simulink model "MagnetoShield_PolePlacement_DUE"  (R2019a)
settings: Solver=FixedStepAuto  StartTime=0.0  StopTime=15  RelTol=1e-3  EnableMultiTasking=on
undefined symbols (not defined in the file): A, B, C, DiscIntNeverNeededParam, i0, K, L, sigbuilder_block, Ts, u0, y0
libraries: MagnetoLibrary x3
settings Model: SimulationMode=external  ExtModeTrigDuration=2  Creator=jakub  LastModifiedBy=jakub
settings OptimizationCC: EnhancedBackFolding=on  PassReuseOutputArgsAs=Individual arguments  MaxStackSize=64  OptimizeBlockOrder=speed  DifferentSizesBufferReuse=on  OptimizationCustomize=off
settings DebuggingCC: ParameterTunabilityLossMsg=error
settings HardwareCC: ProdBitPerPointer=32  ProdBitPerSizeT=32  ProdBitPerPtrDiffT=32  ProdLargestAtomicInteger=Long  ProdLargestAtomicFloat=Double  ProdWordSize=32  ProdHWDeviceType=ARM Compatible->ARM Cortex
settings SFSimCC: MATLABDynamicMemAlloc=off
settings RTWCC: SystemTargetFile=ert.tlc  HardwareBoard=Arduino Due  TLCOptions=-aInlineSetEventsForThisBaseRateFcn=TLC_FALSE -aSuppressMultiTaskScheduler=TLC_FALSE -aRateBasedStepFcn=1  TemplateMakefile=ert_default_tmf  GenerateReport=on  Toolchain=Arduino ARM  BuildConfiguration=Faster Runs  IncludeHyperlinkInReport=on  LaunchReport=on  GenerateTraceInfo=on  GenerateTraceReport=on  GenerateTraceReportSl=on  GenerateTraceReportSf=on  GenerateTraceReportEml=on
settings CodeAppCC: ForceParamTrailComments=on  IgnoreCustomStorageClasses=off  OperatorAnnotations=on  SimulinkDataObjDesc=on  SFDataObjDesc=on  InsertBlockDesc=on
settings ERTTargetCC: SupportContinuousTime=on  SupportVariableSizeSignals=on  ExtModeStaticAllocSize=24576

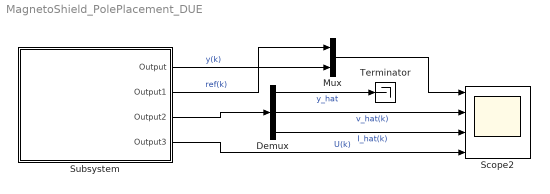
== system MagnetoShield_PolePlacement_DUE ==
  Demux : Demux  Outputs=3
  Mux : Mux  Inputs=2
  Scope2 : Scope  NumInputPorts=4
  Subsystem : Subsystem
  Terminator : Terminator
  wires:
  Subsystem/2(Output1) -> Mux/1  "ref(k)"
  Subsystem/1(Output) -> Mux/2  "y(k)"
  Subsystem/3(Output2) -> Demux/1
  Subsystem/4(Output3) -> Scope2/4  "U(k)"
  Demux/2 -> Scope2/2  "v_hat(k)"
  Demux/3 -> Scope2/3  "I_hat(k)"
  Mux/1 -> Scope2/1
  Demux/1 -> Terminator/1  "y_hat"

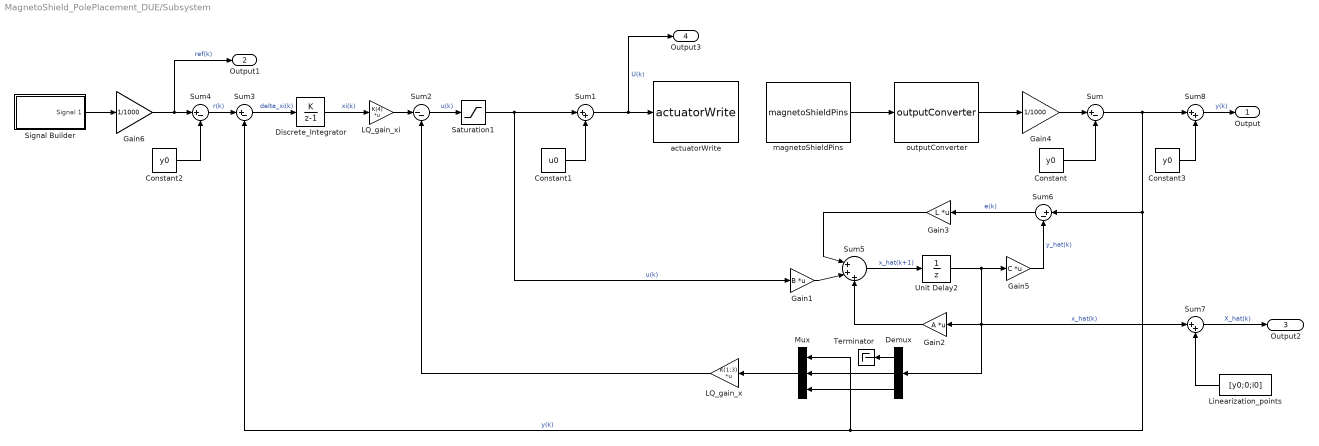
== system MagnetoShield_PolePlacement_DUE/Subsystem ==
  Constant : Constant  Value=y0
  Constant1 : Constant  Value=u0
  Constant2 : Constant  Value=y0
  Constant3 : Constant  Value=y0
  Demux : Demux  Outputs=3
  Discrete_Integrator : DiscreteIntegrator  IntegratorMethod=Accumulation: Forward Euler  SampleTime=Ts  UpperSaturationLimit=1  LowerSaturationLimit=-1  ICPrevOutput=DiscIntNeverNeededParam  ICPrevScaledInput=DiscIntNeverNeededParam
  Gain1 : Gain  Gain=B  Multiplication=Matrix(K*u)
  Gain2 : Gain  Gain=A  Multiplication=Matrix(K*u)
  Gain3 : Gain  Gain=L  Multiplication=Matrix(K*u)
  Gain4 : Gain  Gain=1/1000
  Gain5 : Gain  Gain=C  Multiplication=Matrix(K*u)
  Gain6 : Gain  Gain=1/1000
  LQ_gain_x : Gain  Gain=K(1:3)  Multiplication=Matrix(K*u)
  LQ_gain_xi : Gain  Gain=K(4)  Multiplication=Matrix(K*u)
  Linearization_points : Constant  Value=[y0;0;i0]
  Mux : Mux  Inputs=3
  Saturation1 : Saturate  UpperLimit=10-u0  LowerLimit=0-u0
  Signal Builder : Subsystem  Tag=STV Subsys  LoadFcn=sigbuilder_block('load');  StartFcn=sigbuilder_block('start');  StopFcn=sigbuilder_block('stop');  ClipboardFcn=sigbuilder_block('clipboard');  mask(Sigbuilder block){tuvar=[0:10]}
      mask help: Simulink:masks:SigbuilderBlock_MD
      mask init:
      | if ~strcmp(get_param(bdroot(gcbh),'SimulationStatus'),'stopped') tuvar = sigbuilder_block('maskInit'); end
      settings: CopyFcn=sigbuilder_block('copy');  DeleteFcn=sigbuilder_block('delete');  ModelCloseFcn=sigbuilder_block('modelClose');  PreSaveFcn=sigbuilder_block('preSave');  PauseFcn=sigbuilder_block('pause');  ContinueFcn=sigbuilder_block('continue');  NameChangeFcn=sigbuilder_block('namechange');  OpenFcn=sigbuilder_block('open',[434.4 169.8 550.8 400.2 ]);  CloseFcn=sigbuilder_block('close');
      mask Display: plot(0, 0, 100, 100,[2, 2, 32, 32, 2], [68, 8, 8, 68, 68],[32, 2], [38, 38], [32, 19, 2],[53, 60, 44], [32, 17, 17, 2],[16, 16, 31, 31]);txt = getActiveGroup(gcbh);text(2, 100, txt,'verticalAlignment', 'top');
  Sum{,3..4,6} (4 alike) : Sum  Inputs=|+-
  Sum1 : Sum  Inputs=|++
  Sum2 : Sum  Inputs=|--
  Sum5 : Sum  Inputs=|+++
  Sum7 : Sum  Inputs=|++
  Sum8 : Sum  Inputs=|++
  Terminator : Terminator
  Unit Delay2 : UnitDelay  InitialCondition=[0.017-y0;0;0-i0]  SampleTime=-1  HasFrameUpgradeWarning=on
  actuatorWrite : MagnetoLibrary/actuatorWrite  Board=DUE  Units=Volts
      settings: SourceProductName=AutomationShield
  magnetoShieldPins : MagnetoLibrary/magnetoShieldPins  PIN=Hall sensor pin (A3)  sampling=Ts
      settings: SourceProductName=AutomationShield
  outputConverter : MagnetoLibrary/outputConverter  BoardType=DUE  Units=Position  Pos=Distance  Dconst1=3.233100  Dconst2=0.220571  ADCmin_UNO=27  ADCmax_UNO=776  ADCmin_DUE=100  ADCmax_DUE=2315  ChackBox=off  VoltGain=4  CurrGain=33.333333  Parameter13=on
      settings: SourceProductName=AutomationShield
  Output : Outport
  Output1 : Outport  Port=2
  Output2 : Outport  Port=3
  Output3 : Outport  Port=4
  wires:
  Sum6/1 -> Gain3/1  "e(k)"
  Gain1/1 -> Sum5/2
  Constant1/1 -> Sum1/2
  Constant/1 -> Sum/2
  Unit Delay2/1 -> Gain5/1, Demux/1, Sum7/1, Gain2/1  "x_hat(k)"
  LQ_gain_xi/1 -> Sum2/1
  Gain5/1 -> Sum6/2  "y_hat(k)"
  Gain3/1 -> Sum5/1
  Gain2/1 -> Sum5/3
  outputConverter/1 -> Gain4/1
  Sum4/1 -> Sum3/1  "r(k)"
  Sum2/1 -> Saturation1/1  "u(k)"
  Sum7/1 -> Output2/1  "X_hat(k)"
  Sum1/1 -> actuatorWrite/1, Output3/1  "U(k)"
  Sum3/1 -> Discrete_Integrator/1  "delta_xi(k)"
  Constant2/1 -> Sum4/2
  LQ_gain_x/1 -> Sum2/2
  Sum5/1 -> Unit Delay2/1  "x_hat(k+1)"
  Gain4/1 -> Sum/1
  Saturation1/1 -> Sum1/1, Gain1/1  "u(k)"
  Discrete_Integrator/1 -> LQ_gain_xi/1  "xi(k)"
  Sum/1 -> Sum8/1, Sum6/1, Mux/1, Sum3/2  "y(k)"
  Linearization_points/1 -> Sum7/2
  Gain6/1 -> Output1/1, Sum4/1  "ref(k)"
  Signal Builder/1(Signal 1) -> Gain6/1
  Constant3/1 -> Sum8/2
  Sum8/1 -> Output/1  "y(k)"
  magnetoShieldPins/1 -> outputConverter/1
  Mux/1 -> LQ_gain_x/1
  Demux/2 -> Mux/2
  Demux/3 -> Mux/3
  Demux/1 -> Terminator/1

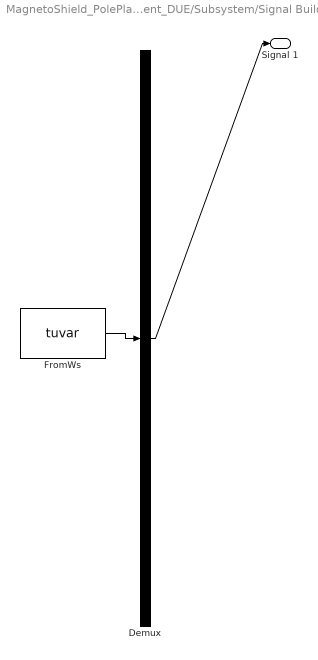
== system MagnetoShield_PolePlacement_DUE/Subsystem/Signal Builder ==
  Demux : Demux  Tag=STV Demux  Outputs=1
  FromWs : FromWorkspace  Tag=STV FromWs  VariableName=tuvar  SampleTime=0
      SigBuilderData=|
      | common.afterFinalStr = 'Extrapolate'
      | common.sampleTime = 0
      | dataSet.timeRange = [0 15]
      | dataSet.name = 'Group 1'
      | sbobj.Groups.Name = 'Group 1'
      | sbobj.Groups.Signals.Name = 'Signal 1'
      | sbobj.Groups.Signals.XData = [0 2 2 4 4 6 6 8 10 12 14 14 15]
      | sbobj.Groups.Signals.YData = [15.5 15.5 14 14 12.5 12.5 14.5 14.5 17 12 14.5 17 17]
      | sbobj.Groups.TimeRange = [0 15]
  Signal 1 : Outport  Tag=STV Outport
  wires:
  FromWs/1 -> Demux/1
  Demux/1 -> Signal 1/1
